simulink model "ex2b2"  (R2020a)
settings: Solver=VariableStepAuto  StartTime=0.0  StopTime=500  RelTol=1e-3
libraries: simulink x2
settings Model: Creator=mumun  LastModifiedBy=mumun

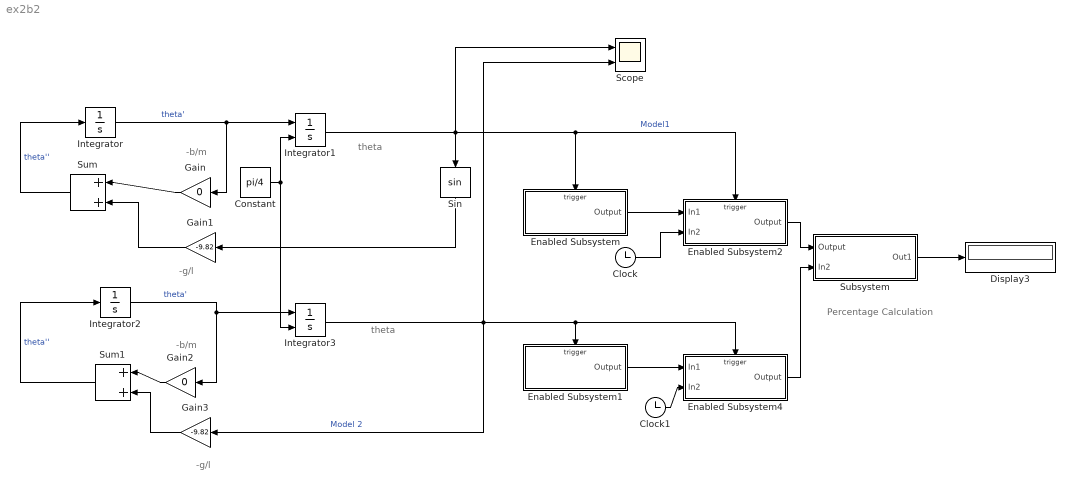
== system ex2b2 ==
  note: Percentage Calculation
  note: -g/l
  note: theta
  note: -g/l
  note: -b/m
  note: -b/m
  note: theta
  Clock : Clock
  Clock1 : Clock
  Constant : Constant  Value=pi/4
  Display3 : Display
  Enabled Subsystem : Subsystem  TreatAsAtomicUnit=on
  Enabled Subsystem1 : Subsystem  TreatAsAtomicUnit=on
  Enabled Subsystem2 : Subsystem  TreatAsAtomicUnit=on
  Enabled Subsystem4 : Subsystem  TreatAsAtomicUnit=on
  Gain : Gain  Gain=0
  Gain1 : Gain  Gain=-9.82
  Gain2 : Gain  Gain=0
  Gain3 : Gain  Gain=-9.82
  Integrator : Integrator
  Integrator1 : Integrator  InitialConditionSource=external
  Integrator2 : Integrator
  Integrator3 : Integrator  InitialConditionSource=external
  Scope : Scope  NumInputPorts=2
  Sin : Trigonometry
  Subsystem : Subsystem
  Sum : Sum  Inputs=|++
  Sum1 : Sum  Inputs=|++
  wires:
  Integrator/1 -> Gain/1, Integrator1/1  "theta'"
  Sin/1 -> Gain1/1
  Gain/1 -> Sum/1
  Gain1/1 -> Sum/2
  Sum/1 -> Integrator/1  "theta''"
  Sum1/1 -> Integrator2/1  "theta''"
  Constant/1 -> Integrator3/2, Integrator1/2
  Gain2/1 -> Sum1/1
  Gain3/1 -> Sum1/2
  Integrator2/1 -> Gain2/1, Integrator3/1  "theta'"
  Integrator3/1 -> Scope/2, Enabled Subsystem4/Trigger, Enabled Subsystem1/Trigger, Gain3/1  "Model 2"
  Integrator1/1 -> Enabled Subsystem2/Trigger, Enabled Subsystem/Trigger, Sin/1, Scope/1  "Model1"
  Enabled Subsystem2/1(Output) -> Subsystem/1(Output)
  Enabled Subsystem1/1(Output) -> Enabled Subsystem4/1(In1)
  Enabled Subsystem4/1(Output) -> Subsystem/2(In2)
  Enabled Subsystem/1(Output) -> Enabled Subsystem2/1(In1)
  Clock/1 -> Enabled Subsystem2/2(In2)
  Clock1/1 -> Enabled Subsystem4/2(In2)
  Subsystem/1(Out1) -> Display3/1

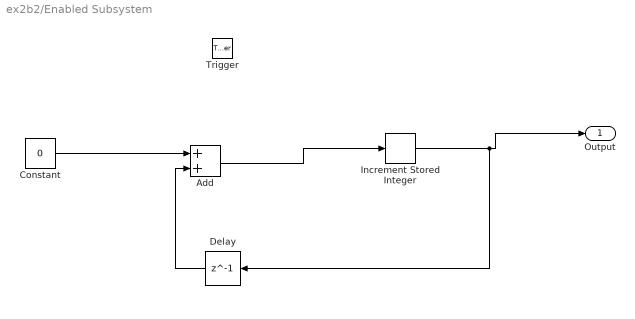
== system ex2b2/Enabled Subsystem ==
  Trigger : TriggerPort  VariantControl=Variant  PortDimensions=1
  Add : Sum
  Constant : Constant  Value=0
  Delay : Delay  DelayLength=1
  Increment Stored Integer : simulink/Additional Math & Discrete/Additional Math: Increment - Decrement/Increment Stored Integer
  Output : Outport
  wires:
  Constant/1 -> Add/1
  Add/1 -> Increment Stored Integer/1
  Increment Stored Integer/1 -> Delay/1, Output/1
  Delay/1 -> Add/2

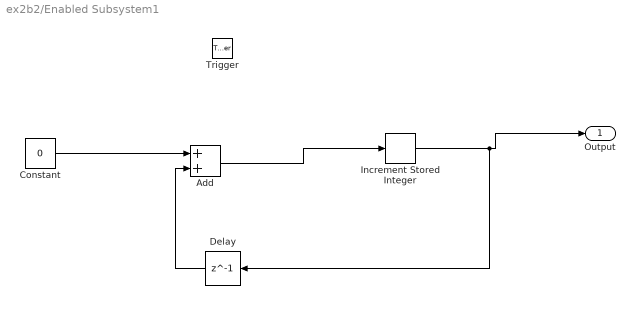
== system ex2b2/Enabled Subsystem1 ==
  Trigger : TriggerPort  VariantControl=Variant  PortDimensions=1
  Add : Sum
  Constant : Constant  Value=0
  Delay : Delay  DelayLength=1
  Increment Stored Integer : simulink/Additional Math & Discrete/Additional Math: Increment - Decrement/Increment Stored Integer
  Output : Outport
  wires:
  Constant/1 -> Add/1
  Add/1 -> Increment Stored Integer/1
  Increment Stored Integer/1 -> Delay/1, Output/1
  Delay/1 -> Add/2

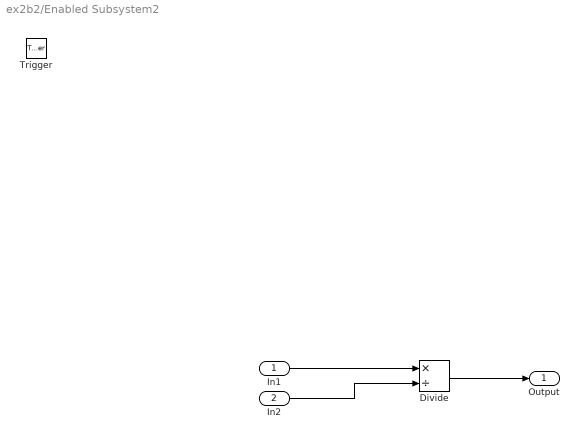
== system ex2b2/Enabled Subsystem2 ==
  In1 : Inport
  In2 : Inport  Port=2
  Trigger : TriggerPort  VariantControl=Variant  PortDimensions=1
  Divide : Product  Inputs=*/
  Output : Outport
  wires:
  In1/1 -> Divide/1
  Divide/1 -> Output/1
  In2/1 -> Divide/2

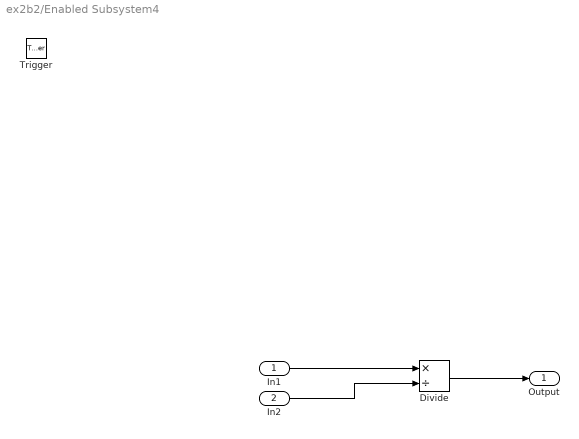
== system ex2b2/Enabled Subsystem4 ==
  In1 : Inport
  In2 : Inport  Port=2
  Trigger : TriggerPort  VariantControl=Variant  PortDimensions=1
  Divide : Product  Inputs=*/
  Output : Outport
  wires:
  In1/1 -> Divide/1
  Divide/1 -> Output/1
  In2/1 -> Divide/2

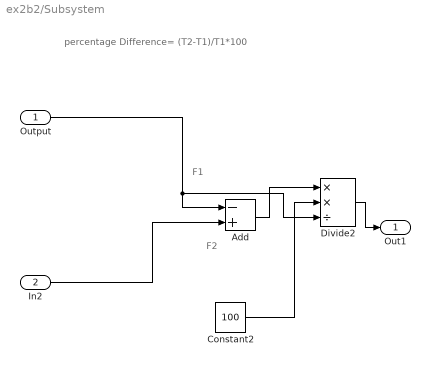
== system ex2b2/Subsystem ==
  note: F2
  note: F1
  note: percentage Difference= (T2-T1)/T1*100
  Output : Inport
  In2 : Inport  Port=2
  Add : Sum  Inputs=-+
  Constant2 : Constant  Value=100
  Divide2 : Product  Inputs=**/
  Out1 : Outport
  wires:
  In2/1 -> Add/2
  Add/1 -> Divide2/1
  Constant2/1 -> Divide2/2
  Output/1 -> Add/1, Divide2/3
  Divide2/1 -> Out1/1
